simulink model "NetrAI_Telemedicine_Model"  (R2026a)
settings: Solver=VariableStepDiscrete  StopTime=simulationDuration
model workspace (MAT data in the model file):
  acquisitionQueueCapacity = 100001
  acquisitionTime = 45
  aiInferenceTime = 3.5
  aiQueueCapacity = 100001
  autoClearRate = 0.9077
  bandwidthMbps = 1
  clinicianCount = 1
  imageSizeMB = 3.5
  imagesPerPatient = 2
  interarrivalTime = 72
  operatingHoursPerDay = 8
  qualityRejectRate = 0.1
  recaptureQueueCapacity = 100001
  recaptureTime = 120
  referRate = 0.08
  reviewQueueCapacity = 100001
  reviewTimePerPatient = 30
  simulationDuration = 7200000
  totalPatients = 100000
  uncertainRate = 0.0123
  uploadQueueCapacity = 100001
  uploadTime = 56
  workingDays = 250
undefined symbols (not defined in the file or in its folder): m, n
Description:
  | NetrAI district telemedicine digital twin: 100,000 patients/year, recapture, bandwidth, AI, and review queues.
settings Model: Creator=ovoabhik  LastModifiedBy=ovoabhik

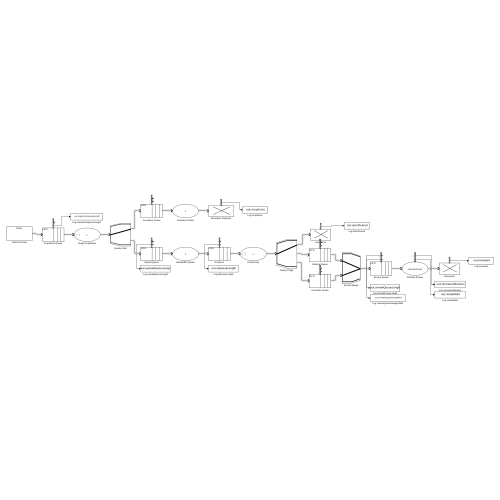
[thumbnail: Simulink's stored preview of the top-level diagram]
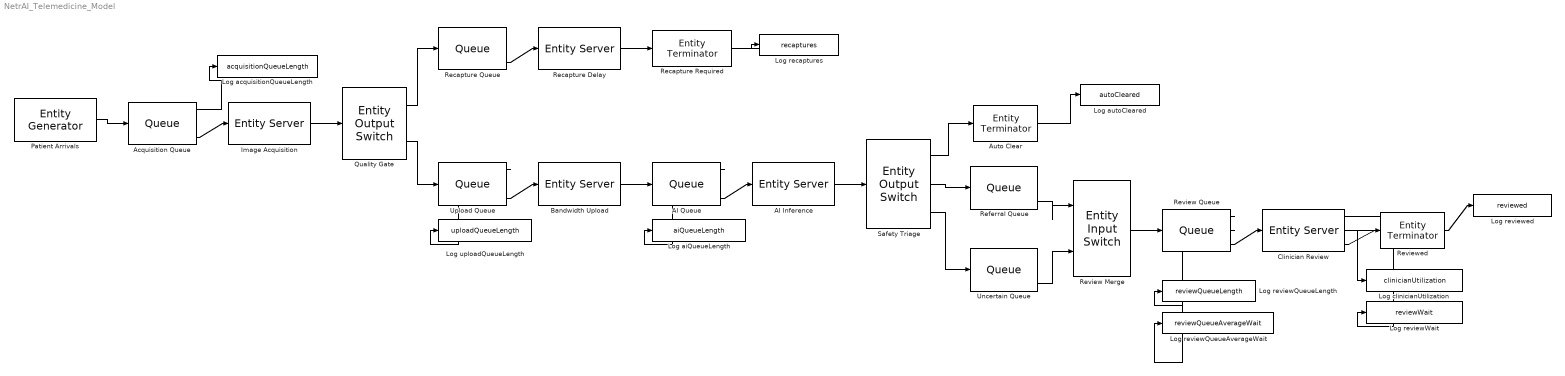
== system NetrAI_Telemedicine_Model ==
  AI Inference : EntityServer  InputPortMessageModes=m  OutputPortMessageModes=m  Capacity=1  ServiceTimeValue=aiInferenceTime  ServiceCompleteAction=|
      | u = rand();
      | if u < autoClearRate
      |     entity.Attribute1 = 1;
      | elseif u < autoClearRate + referRate
      |     entity.Attribute1 = 2;
      | else
      |     entity.Attribute1 = 3;
      | end
  AI Queue : Queue  InputPortMessageModes=m  OutputPortMessageModes=n,n,m  Capacity=aiQueueCapacity  NumberEntitiesInBlock=on  AverageWait=on
      settings: OutputPortMap=o1,o2,o5
  Acquisition Queue : Queue  InputPortMessageModes=m  OutputPortMessageModes=n,n,m  Capacity=acquisitionQueueCapacity  NumberEntitiesInBlock=on  AverageWait=on
      settings: OutputPortMap=o1,o2,o5
  Auto Clear : EntityTerminator  InputPortMessageModes=m  NumberEntitiesArrived=on
      settings: OutputPortMap=o0
  Bandwidth Upload : EntityServer  InputPortMessageModes=m  OutputPortMessageModes=m  Capacity=1  ServiceTimeValue=uploadTime
  Clinician Review : EntityServer  InputPortMessageModes=m  OutputPortMessageModes=n,n,m  Capacity=clinicianCount  ServiceTimeValue=reviewTimePerPatient  AverageWait=on  Utilization=on
      settings: OutputPortMap=o4,o5,o9
  Image Acquisition : EntityServer  InputPortMessageModes=m  OutputPortMessageModes=m  Capacity=1  ServiceTimeValue=acquisitionTime  ServiceCompleteAction=|
      | if rand() < qualityRejectRate
      |     entity.Attribute1 = 1;
      | else
      |     entity.Attribute1 = 2;
      | end
  Log acquisitionQueueLength : ToWorkspace  VariableName=acquisitionQueueLength  SaveFormat=Timeseries  SampleTime=-1
  Log aiQueueLength : ToWorkspace  VariableName=aiQueueLength  SaveFormat=Timeseries  SampleTime=-1
  Log autoCleared : ToWorkspace  VariableName=autoCleared  SaveFormat=Timeseries  SampleTime=-1
  Log clinicianUtilization : ToWorkspace  VariableName=clinicianUtilization  SaveFormat=Timeseries  SampleTime=-1
  Log recaptures : ToWorkspace  VariableName=recaptures  SaveFormat=Timeseries  SampleTime=-1
  Log reviewQueueAverageWait : ToWorkspace  VariableName=reviewQueueAverageWait  SaveFormat=Timeseries  SampleTime=-1
  Log reviewQueueLength : ToWorkspace  VariableName=reviewQueueLength  SaveFormat=Timeseries  SampleTime=-1
  Log reviewWait : ToWorkspace  VariableName=reviewWait  SaveFormat=Timeseries  SampleTime=-1
  Log reviewed : ToWorkspace  VariableName=reviewed  SaveFormat=Timeseries  SampleTime=-1
  Log uploadQueueLength : ToWorkspace  VariableName=uploadQueueLength  SaveFormat=Timeseries  SampleTime=-1
  Patient Arrivals : EntityGenerator  OutputPortMessageModes=m  Period=interarrivalTime  AttributeInitialValue=2  EntityType=Structured  EntityTypeName=Entity
  Quality Gate : EntityOutputSwitch  InputPortMessageModes=m  OutputPortMessageModes=m,m  SwitchingCriterion=From attribute  SwitchAttributeName=Attribute1
  Recapture Delay : EntityServer  InputPortMessageModes=m  OutputPortMessageModes=m  Capacity=1  ServiceTimeValue=recaptureTime
  Recapture Queue : Queue  InputPortMessageModes=m  OutputPortMessageModes=n,n,m  Capacity=recaptureQueueCapacity  NumberEntitiesInBlock=on  AverageWait=on
      settings: OutputPortMap=o1,o2,o5
  Recapture Required : EntityTerminator  InputPortMessageModes=m  NumberEntitiesArrived=on
      settings: OutputPortMap=o0
  Referral Queue : Queue  InputPortMessageModes=m  OutputPortMessageModes=n,n,m  Capacity=reviewQueueCapacity  NumberEntitiesInBlock=on  AverageWait=on
      settings: OutputPortMap=o1,o2,o5
  Review Merge : EntityInputSwitch  InputPortMessageModes=m,m  OutputPortMessageModes=m
  Review Queue : Queue  InputPortMessageModes=m  OutputPortMessageModes=n,n,m  Capacity=reviewQueueCapacity  NumberEntitiesInBlock=on  AverageWait=on
      settings: OutputPortMap=o1,o2,o5
  Reviewed : EntityTerminator  InputPortMessageModes=m  NumberEntitiesArrived=on
      settings: OutputPortMap=o0
  Safety Triage : EntityOutputSwitch  InputPortMessageModes=m  OutputPortMessageModes=m,m,m  NumberOutputPorts=3  SwitchingCriterion=From attribute  SwitchAttributeName=Attribute1
      settings: OutputPortMap=o0,o1,o2
  Uncertain Queue : Queue  InputPortMessageModes=m  OutputPortMessageModes=n,n,m  Capacity=reviewQueueCapacity  NumberEntitiesInBlock=on  AverageWait=on
      settings: OutputPortMap=o1,o2,o5
  Upload Queue : Queue  InputPortMessageModes=m  OutputPortMessageModes=n,n,m  Capacity=uploadQueueCapacity  NumberEntitiesInBlock=on  AverageWait=on
      settings: OutputPortMap=o1,o2,o5
  wires:
  Patient Arrivals/1 -> Acquisition Queue/1
  Acquisition Queue/3 -> Image Acquisition/1
  Image Acquisition/1 -> Quality Gate/1
  Quality Gate/1 -> Recapture Queue/1
  Recapture Queue/3 -> Recapture Delay/1
  Recapture Delay/1 -> Recapture Required/1
  Quality Gate/2 -> Upload Queue/1
  Upload Queue/3 -> Bandwidth Upload/1
  Bandwidth Upload/1 -> AI Queue/1
  AI Queue/3 -> AI Inference/1
  AI Inference/1 -> Safety Triage/1
  Safety Triage/1 -> Auto Clear/1
  Safety Triage/2 -> Referral Queue/1
  Safety Triage/3 -> Uncertain Queue/1
  Referral Queue/3 -> Review Merge/1
  Uncertain Queue/3 -> Review Merge/2
  Review Merge/1 -> Review Queue/1
  Review Queue/3 -> Clinician Review/1
  Clinician Review/3 -> Reviewed/1
  Auto Clear/1 -> Log autoCleared/1
  Reviewed/1 -> Log reviewed/1
  Recapture Required/1 -> Log recaptures/1
  Clinician Review/2 -> Log clinicianUtilization/1
  Clinician Review/1 -> Log reviewWait/1
  Acquisition Queue/1 -> Log acquisitionQueueLength/1
  Upload Queue/1 -> Log uploadQueueLength/1
  AI Queue/1 -> Log aiQueueLength/1
  Review Queue/1 -> Log reviewQueueLength/1
  Review Queue/2 -> Log reviewQueueAverageWait/1
